simulink model "HoppingModel_Position"  (R2020a)
settings: Solver=FixedStepAuto  StartTime=0.0  StopTime=2  FixedStep=0.001  RelTol=1e-3
undefined symbols (not defined in the file or in its folder): chi_0, desired_energy, desired_energy2, desired_energy3, desired_energy4, desired_energy5, desired_energy6, desired_energy7, desired_energy8, g, H, H2, H3, H4, H5, H6, H7, H8, I1, I2, ini_theta1, ini_theta1_d, ini_theta2, ini_theta2_d, ini_w, ini_w_d, ini_x0, ini_x0_d, ini_x1, ini_x1_d, ini_x2, ini_x2_d, ini_y0, ini_y0_d, ini_y1, ini_y1_d, ini_y2, ini_y2_d, M1, M2, r1, r2, start_1, start_2, start_3, T2_change, T3_change, T4_change, T5_change, T6_change, T7_change, T8_change, x2_desired_1, x2_desired_2, x2_desired_3
settings Model: Creator=fabia  LastModifiedBy=fabia
settings DataIOCC: ReturnWorkspaceOutputs=off

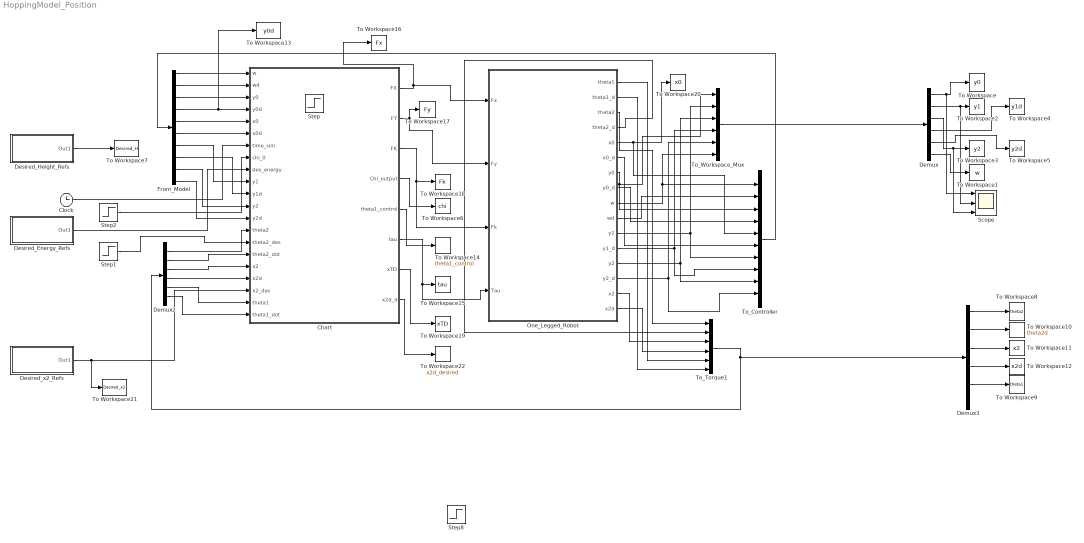
== system HoppingModel_Position ==
  Chart : Stateflow chart  TreatAsAtomicUnit=on
      settings: PortSchema="{\"entries\":[{\"content\":{\"sides\":[{\"content\":{\"connectorIds\":[\"In1\",\"In2\",\"In3\",\"In4\",\"In5\",\"In6\",\"In7\",\"In8\",\"In9\",\"In10\",\"In11\",\"In12\",\"In13\",\"In14\",\"In15\",\"In16\",\"In17\",\"In18\",\"In19\",\"In20\",\"In21\"]},\"type\":\"ConnectorPlacement.EquallySpacedRectSide\",\"uuid\":\"d60879a0-12a6-4ea9-8b3c-a4e8171fc461\"},{\"content\":{\"connectorIds\":[\"Out2\",\"Out1\",\"Out3\",\"Out4\",\"Out5\",\"Out6\",\"Out7\",\"Out8\"],\"side\":\"RIGHT\"},\"type\":\"ConnectorPlacement.EquallySpacedRectSide\",\"uuid\":\"e7f8c78b-f9da-45a1-b210-b73b1fe065f3\"},{\"content\":{\"connectorIds\":[],\"side\":\"TOP\"},\"type\":\"ConnectorPlacement.EquallySpacedRectSide\",\"uuid\":\"a7cfd386-52b0-4dd7-827b-34f43a49e5d2\"}]},\"type\":\"ConnectorPlacement.EquallySpacedConnector\",\"uuid\":\"c0fe03cd-cdd0-4cdb-8340-587840dec8d6\"}],\"packageUris\":[\"http://schema.mathworks.com/mf0/Connector/19700101\"],\"version\":\"1.0\"}"
  Clock : Clock
  Demux : Demux  Outputs=6
  Demux2 : Demux  Outputs=6
  Demux3 : Demux  Outputs=6
  Desired_Energy_Refs : Subsystem
  Desired_Height_Refs : Subsystem
  Desired_x2_Refs : Subsystem
  From_Model : Demux  Outputs=10
  One_Legged_Robot : Subsystem
  Scope : Scope  NumInputPorts=3
  Step : Step  Time=0  After=0  SampleTime=0
  Step1 : Step  Time=0  After=0  SampleTime=0
  Step2 : Step  Time=0  After=chi_0  SampleTime=0
  Step8 : Step  Time=T2_change  After=H2  SampleTime=0
  To Workspace : ToWorkspace  VariableName=y0  SaveFormat=Timeseries  SampleTime=-1
      settings: Save2DSignal=2-D array (concatenate along first dimension)
  To Workspace1 : ToWorkspace  VariableName=w  SaveFormat=Timeseries  SampleTime=-1
      settings: Save2DSignal=2-D array (concatenate along first dimension)
  To Workspace10 : ToWorkspace  VariableName=theta2d  SaveFormat=Timeseries  SampleTime=-1
      settings: Save2DSignal=2-D array (concatenate along first dimension)
  To Workspace11 : ToWorkspace  VariableName=x2  SaveFormat=Timeseries  SampleTime=-1
      settings: Save2DSignal=2-D array (concatenate along first dimension)
  To Workspace12 : ToWorkspace  VariableName=x2d  SaveFormat=Timeseries  SampleTime=-1
      settings: Save2DSignal=2-D array (concatenate along first dimension)
  To Workspace13 : ToWorkspace  VariableName=y0d  SaveFormat=Timeseries  SampleTime=-1
  To Workspace14 : ToWorkspace  VariableName=theta1_control  SaveFormat=Timeseries  SampleTime=-1
      settings: Save2DSignal=2-D array (concatenate along first dimension)
  To Workspace15 : ToWorkspace  VariableName=tau  SaveFormat=Timeseries  SampleTime=-1
      settings: Save2DSignal=2-D array (concatenate along first dimension)
  To Workspace16 : ToWorkspace  VariableName=Fx  SaveFormat=Timeseries  SampleTime=-1
      settings: Save2DSignal=2-D array (concatenate along first dimension)
  To Workspace17 : ToWorkspace  VariableName=Fy  SaveFormat=Timeseries  SampleTime=-1
      settings: Save2DSignal=2-D array (concatenate along first dimension)
  To Workspace18 : ToWorkspace  VariableName=Fk  SaveFormat=Timeseries  SampleTime=-1
      settings: Save2DSignal=2-D array (concatenate along first dimension)
  To Workspace19 : ToWorkspace  VariableName=xTD  SaveFormat=Timeseries  SampleTime=-1
      settings: Save2DSignal=2-D array (concatenate along first dimension)
  To Workspace2 : ToWorkspace  VariableName=y1  SaveFormat=Timeseries  SampleTime=-1
      settings: Save2DSignal=2-D array (concatenate along first dimension)
  To Workspace20 : ToWorkspace  VariableName=x0  SaveFormat=Timeseries  SampleTime=-1
      settings: Save2DSignal=2-D array (concatenate along first dimension)
  To Workspace21 : ToWorkspace  VariableName=Desired_x2  SaveFormat=Timeseries  SampleTime=-1
  To Workspace22 : ToWorkspace  VariableName=x2d_desired  SaveFormat=Timeseries  SampleTime=-1
      settings: Save2DSignal=2-D array (concatenate along first dimension)
  To Workspace3 : ToWorkspace  VariableName=y2  SaveFormat=Timeseries  SampleTime=-1
      settings: Save2DSignal=2-D array (concatenate along first dimension)
  To Workspace4 : ToWorkspace  VariableName=y1d  SaveFormat=Timeseries  SampleTime=-1
      settings: Save2DSignal=2-D array (concatenate along first dimension)
  To Workspace5 : ToWorkspace  VariableName=y2d  SaveFormat=Timeseries  SampleTime=-1
      settings: Save2DSignal=2-D array (concatenate along first dimension)
  To Workspace6 : ToWorkspace  VariableName=chi  SaveFormat=Timeseries  SampleTime=-1
      settings: Save2DSignal=2-D array (concatenate along first dimension)
  To Workspace7 : ToWorkspace  VariableName=Desired_H  SaveFormat=Timeseries  SampleTime=-1
  To Workspace8 : ToWorkspace  VariableName=theta2  SaveFormat=Timeseries  SampleTime=-1
      settings: Save2DSignal=2-D array (concatenate along first dimension)
  To Workspace9 : ToWorkspace  VariableName=theta1  SaveFormat=Timeseries  SampleTime=-1
      settings: Save2DSignal=2-D array (concatenate along first dimension)
  To_Controller : Mux  Inputs=10
  To_Torque1 : Mux  Inputs=6
  To_Workspace_Mux : Mux  Inputs=6
  wires:
  One_Legged_Robot/11(y1) -> To_Controller/7, To_Workspace_Mux/2
  One_Legged_Robot/13(y2) -> To_Controller/9, To_Workspace_Mux/3
  One_Legged_Robot/7(y0) -> To_Controller/3, To_Workspace_Mux/1
  One_Legged_Robot/5(x0) -> To Workspace20/1, To_Controller/5
  One_Legged_Robot/10(wd) -> To_Controller/2
  One_Legged_Robot/8(y0_d) -> To_Controller/4
  Chart/2(FX) -> One_Legged_Robot/1(Fx), To Workspace16/1
  Chart/1(FY) -> One_Legged_Robot/2(Fy), To Workspace17/1
  Chart/3(FK) -> To Workspace18/1, One_Legged_Robot/3(Fk)
  One_Legged_Robot/9(w) -> To_Workspace_Mux/6, To_Controller/1
  Clock/1 -> Chart/7(time_sim)
  Step2/1 -> Chart/8(chi_0)
  One_Legged_Robot/14(y2_d) -> To_Controller/10, To_Workspace_Mux/5
  Chart/4(Chi_output) -> To Workspace6/1
  One_Legged_Robot/6(x0_d) -> To_Controller/6
  One_Legged_Robot/12(y1_d) -> To_Controller/8, To_Workspace_Mux/4
  One_Legged_Robot/1(theta1) -> To_Torque1/5
  One_Legged_Robot/2(theta1_d) -> To_Torque1/6
  To_Controller/1 -> From_Model/1
  From_Model/1 -> Chart/1(w)
  From_Model/2 -> Chart/2(wd)
  From_Model/3 -> Chart/3(y0)
  From_Model/4 -> To Workspace13/1, Chart/4(y0d)
  From_Model/5 -> Chart/5(x0)
  From_Model/6 -> Chart/6(x0d)
  From_Model/7 -> Chart/10(y1)
  From_Model/8 -> Chart/11(y1d)
  From_Model/9 -> Chart/12(y2)
  From_Model/10 -> Chart/13(y2d)
  To_Workspace_Mux/1 -> Demux/1
  Demux/1 -> Scope/1, To Workspace/1
  Demux/2 -> Scope/2, To Workspace2/1
  Demux/3 -> Scope/3, To Workspace3/1
  Demux/4 -> To Workspace4/1
  Demux/5 -> To Workspace5/1
  Demux/6 -> To Workspace1/1
  Desired_Energy_Refs/1(Out1) -> Chart/9(des_energy)
  Desired_Height_Refs/1(Out1) -> To Workspace7/1
  One_Legged_Robot/3(theta2) -> To_Torque1/1
  One_Legged_Robot/4(theta2_d) -> To_Torque1/2
  One_Legged_Robot/15(x2) -> To_Torque1/3
  One_Legged_Robot/16(x2d) -> To_Torque1/4
  Demux2/1 -> Chart/14(theta2)
  Demux2/2 -> Chart/16(theta2_dot)
  Demux2/3 -> Chart/17(x2)
  Demux2/4 -> Chart/18(x2d)
  To_Torque1/1 -> Demux2/1, Demux3/1
  Chart/5(theta1_control) -> To Workspace14/1
  Step1/1 -> Chart/15(theta2_des)
  Demux3/4 -> To Workspace12/1
  Demux3/1 -> To Workspace8/1
  Demux3/3 -> To Workspace11/1
  Demux3/2 -> To Workspace10/1
  Demux3/5 -> To Workspace9/1
  Demux2/5 -> Chart/20(theta1)
  Demux2/6 -> Chart/21(theta1_dot)
  Chart/6(tau) -> One_Legged_Robot/4(Tau), To Workspace15/1
  Chart/7(xTD) -> To Workspace19/1
  Desired_x2_Refs/1(Out1) -> To Workspace21/1, Chart/19(x2_des)
  Chart/8(x2d_d) -> To Workspace22/1

== system HoppingModel_Position/Desired_Energy_Refs ==
  Add : Sum  Inputs=+-+-+-+-+-+-+-+
  Step1 : Step  Time=T3_change  After=desired_energy2  SampleTime=0
  Step10 : Step  Time=T6_change  After=desired_energy5  SampleTime=0
  Step11 : Step  Time=T6_change  After=desired_energy6  SampleTime=0
  Step12 : Step  Time=T7_change  After=desired_energy6  SampleTime=0
  Step13 : Step  Time=T7_change  After=desired_energy7  SampleTime=0
  Step14 : Step  Time=T8_change  After=desired_energy7  SampleTime=0
  Step15 : Step  Time=T8_change  After=desired_energy8  SampleTime=0
  Step2 : Step  Time=T3_change  After=desired_energy3  SampleTime=0
  Step3 : Step  Time=T4_change  After=desired_energy3  SampleTime=0
  Step4 : Step  Time=0  After=desired_energy  SampleTime=0
  Step5 : Step  Time=T2_change  After=desired_energy  SampleTime=0
  Step6 : Step  Time=T2_change  After=desired_energy2  SampleTime=0
  Step7 : Step  Time=T4_change  After=desired_energy4  SampleTime=0
  Step8 : Step  Time=T5_change  After=desired_energy4  SampleTime=0
  Step9 : Step  Time=T5_change  After=desired_energy5  SampleTime=0
  Out1 : Outport
  wires:
  Step6/1 -> Add/3
  Step4/1 -> Add/1
  Step5/1 -> Add/2
  Add/1 -> Out1/1
  Step1/1 -> Add/4
  Step2/1 -> Add/5
  Step3/1 -> Add/6
  Step7/1 -> Add/7
  Step8/1 -> Add/8
  Step9/1 -> Add/9
  Step10/1 -> Add/10
  Step11/1 -> Add/11
  Step12/1 -> Add/12
  Step13/1 -> Add/13
  Step14/1 -> Add/14
  Step15/1 -> Add/15

== system HoppingModel_Position/Desired_Height_Refs ==
  Add : Sum  Inputs=+-+-+-+-+-+-+-+
  Step1 : Step  Time=T3_change  After=H2  SampleTime=0
  Step10 : Step  Time=T6_change  After=H5  SampleTime=0
  Step11 : Step  Time=T6_change  After=H6  SampleTime=0
  Step12 : Step  Time=T7_change  After=H6  SampleTime=0
  Step13 : Step  Time=T7_change  After=H7  SampleTime=0
  Step14 : Step  Time=T8_change  After=H7  SampleTime=0
  Step15 : Step  Time=T8_change  After=H8  SampleTime=0
  Step2 : Step  Time=T3_change  After=H3  SampleTime=0
  Step3 : Step  Time=T4_change  After=H3  SampleTime=0
  Step4 : Step  Time=0  After=H  SampleTime=0
  Step5 : Step  Time=T2_change  After=H  SampleTime=0
  Step6 : Step  Time=T2_change  After=H2  SampleTime=0
  Step7 : Step  Time=T4_change  After=H4  SampleTime=0
  Step8 : Step  Time=T5_change  After=H4  SampleTime=0
  Step9 : Step  Time=T5_change  After=H5  SampleTime=0
  Out1 : Outport
  wires:
  Step6/1 -> Add/3
  Step4/1 -> Add/1
  Step5/1 -> Add/2
  Add/1 -> Out1/1
  Step1/1 -> Add/4
  Step2/1 -> Add/5
  Step3/1 -> Add/6
  Step7/1 -> Add/7
  Step8/1 -> Add/8
  Step9/1 -> Add/9
  Step10/1 -> Add/10
  Step11/1 -> Add/11
  Step12/1 -> Add/12
  Step13/1 -> Add/13
  Step14/1 -> Add/14
  Step15/1 -> Add/15

== system HoppingModel_Position/Desired_x2_Refs ==
  Add : Sum  Inputs=+-+-+
  Step1 : Step  Time=start_2  After=x2_desired_1  SampleTime=0
  Step2 : Step  Time=start_3  After=x2_desired_2  SampleTime=0
  Step3 : Step  Time=start_3  After=x2_desired_3  SampleTime=0
  Step4 : Step  Time=start_1  After=x2_desired_1  SampleTime=0
  Step6 : Step  Time=start_2  After=x2_desired_2  SampleTime=0
  Out1 : Outport
  wires:
  Step6/1 -> Add/3
  Step4/1 -> Add/1
  Step1/1 -> Add/2
  Add/1 -> Out1/1
  Step2/1 -> Add/4
  Step3/1 -> Add/5

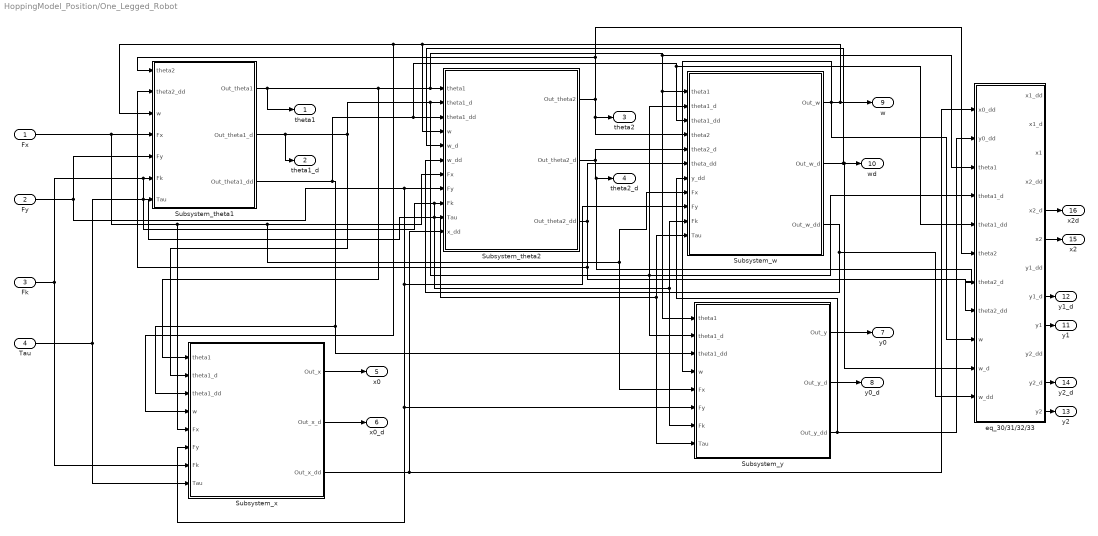
== system HoppingModel_Position/One_Legged_Robot ==
  Fx : Inport
  Fy : Inport  Port=2
  Fk : Inport  Port=3
  Tau : Inport  Port=4
  Subsystem_theta1 : Subsystem
  Subsystem_theta2 : Subsystem
  Subsystem_w : Subsystem
  Subsystem_x : Subsystem
  Subsystem_y : Subsystem
  "eq_30/31/32/33 " : Subsystem
  theta1 : Outport
  theta1_d : Outport  Port=2
  theta2 : Outport  Port=3
  theta2_d : Outport  Port=4
  x0 : Outport  Port=5
  x0_d : Outport  Port=6
  y0 : Outport  Port=7
  y0_d : Outport  Port=8
  w : Outport  Port=9
  wd : Outport  Port=10
  y1 : Outport  Port=11
  y1_d : Outport  Port=12
  y2 : Outport  Port=13
  y2_d : Outport  Port=14
  x2 : Outport  Port=15
  x2d : Outport  Port=16
  wires:
  Subsystem_theta1/1(Out_theta1) -> Subsystem_x/1(theta1), "eq_30/31/32/33 "/3(theta1), Subsystem_y/1(theta1), Subsystem_w/1(theta1), Subsystem_theta2/1(theta1), theta1/1
  Subsystem_theta1/2(Out_theta1_d) -> Subsystem_y/2(theta1_d), "eq_30/31/32/33 "/4(theta1_d), Subsystem_w/2(theta1_d), Subsystem_theta2/2(theta1_d), Subsystem_x/2(theta1_d), theta1_d/1
  Subsystem_x/1(Out_x) -> x0/1
  Subsystem_x/2(Out_x_d) -> x0_d/1
  Subsystem_y/1(Out_y) -> y0/1
  Subsystem_y/2(Out_y_d) -> y0_d/1
  "eq_30/31/32/33 "/9(y1) -> y1/1
  "eq_30/31/32/33 "/8(y1_d) -> y1_d/1
  "eq_30/31/32/33 "/12(y2) -> y2/1
  "eq_30/31/32/33 "/11(y2_d) -> y2_d/1
  Subsystem_w/2(Out_w_d) -> "eq_30/31/32/33 "/10(w_d), wd/1, Subsystem_theta2/5(w_d)
  Subsystem_w/1(Out_w) -> Subsystem_y/4(w), "eq_30/31/32/33 "/9(w), Subsystem_theta2/4(w), Subsystem_x/4(w), Subsystem_theta1/3(w), w/1
  Subsystem_theta2/1(Out_theta2) -> "eq_30/31/32/33 "/6(theta2), Subsystem_theta1/1(theta2), Subsystem_w/4(theta2), theta2/1
  Subsystem_theta2/2(Out_theta2_d) -> Subsystem_w/5(theta2_d), "eq_30/31/32/33 "/7(theta2_d), theta2_d/1
  Subsystem_theta1/3(Out_theta1_dd) -> Subsystem_x/3(theta1_dd), Subsystem_y/3(theta1_dd), "eq_30/31/32/33 "/5(theta1_dd), Subsystem_w/3(theta1_dd), Subsystem_theta2/3(theta1_dd)
  Subsystem_theta2/3(Out_theta2_dd) -> "eq_30/31/32/33 "/8(theta2_dd), Subsystem_theta1/2(theta2_dd), Subsystem_w/6(theta_dd)
  Subsystem_w/3(Out_w_dd) -> "eq_30/31/32/33 "/11(w_dd), Subsystem_theta2/6(w_dd)
  Subsystem_y/3(Out_y_dd) -> "eq_30/31/32/33 "/2(y0_dd), Subsystem_w/7(y_dd)
  Subsystem_x/3(Out_x_dd) -> "eq_30/31/32/33 "/1(x0_dd), Subsystem_theta2/11(x_dd)
  Fx/1 -> Subsystem_x/5(Fx), Subsystem_y/5(Fx), Subsystem_w/8(Fx), Subsystem_theta2/7(Fx), Subsystem_theta1/4(Fx)
  Fy/1 -> Subsystem_w/9(Fy), Subsystem_x/6(Fy), Subsystem_y/6(Fy), Subsystem_theta2/8(Fy), Subsystem_theta1/5(Fy)
  Fk/1 -> Subsystem_x/7(Fk), Subsystem_y/7(Fk), Subsystem_w/10(Fk), Subsystem_theta2/9(Fk), Subsystem_theta1/6(Fk)
  Tau/1 -> Subsystem_x/8(Tau), Subsystem_y/8(Tau), Subsystem_w/11(Tau), Subsystem_theta2/10(Tau), Subsystem_theta1/7(Tau)
  "eq_30/31/32/33 "/6(x2) -> x2/1
  "eq_30/31/32/33 "/5(x2_d) -> x2d/1

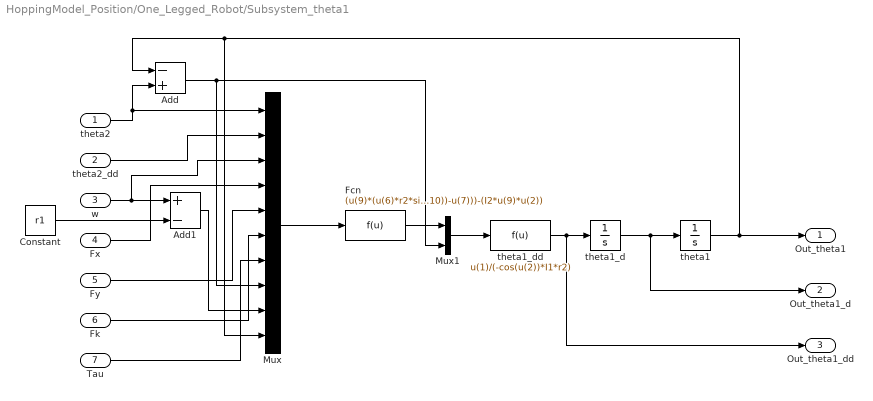
== system HoppingModel_Position/One_Legged_Robot/Subsystem_theta1 ==
  theta2 : Inport
  theta2_dd : Inport  Port=2
  w : Inport  Port=3
  Fx : Inport  Port=4
  Fy : Inport  Port=5
  Fk : Inport  Port=6
  Tau : Inport  Port=7
  Add : Sum  Inputs=-+
  Add1 : Sum  Inputs=+-
  Constant : Constant  Value=r1
  Fcn : Fcn  Expr=(u(9)*(u(6)*r2*sin(u(8))+u(7)))-(r2*cos(u(8))*(r1*u(5)*sin(u(10))-r1*u(4)*cos(u(10))-u(7)))-(I2*u(9)*u(2))
  Mux : Mux  Inputs=10
  Mux1 : Mux  Inputs=2
  theta1 : Integrator  InitialCondition=ini_theta1  UpperSaturationLimit=pi/2  LowerSaturationLimit=-pi/2
  theta1_d : Integrator  InitialCondition=ini_theta1_d  UpperSaturationLimit=pi/2  LowerSaturationLimit=-pi/2
  theta1_dd : Fcn  Expr=u(1)/(-cos(u(2))*I1*r2)
  Out_theta1 : Outport
  Out_theta1_d : Outport  Port=2
  Out_theta1_dd : Outport  Port=3
  wires:
  theta2/1 -> Mux/1, Add/2
  theta1/1 -> Out_theta1/1, Mux/10, Add/1
  w/1 -> Mux/3, Add1/1
  Constant/1 -> Add1/2
  theta2_dd/1 -> Mux/2
  Fx/1 -> Mux/4
  Fy/1 -> Mux/5
  Fk/1 -> Mux/6
  Tau/1 -> Mux/7
  Add/1 -> Mux/8, Mux1/2
  Add1/1 -> Mux/9
  Mux/1 -> Fcn/1
  Fcn/1 -> Mux1/1
  Mux1/1 -> theta1_dd/1
  theta1_dd/1 -> Out_theta1_dd/1, theta1_d/1
  theta1_d/1 -> Out_theta1_d/1, theta1/1

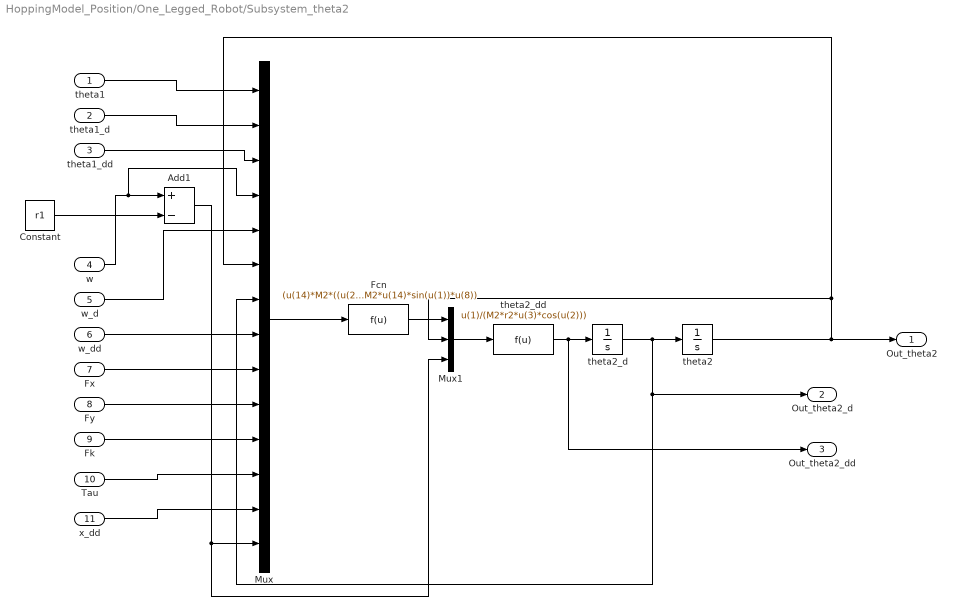
== system HoppingModel_Position/One_Legged_Robot/Subsystem_theta2 ==
  theta1 : Inport
  theta1_d : Inport  Port=2
  theta1_dd : Inport  Port=3
  w : Inport  Port=4
  w_d : Inport  Port=5
  w_dd : Inport  Port=6
  Fx : Inport  Port=7
  Fy : Inport  Port=8
  Fk : Inport  Port=9
  Tau : Inport  Port=10
  x_dd : Inport  Port=11
  Add1 : Sum  Inputs=+-
  Constant : Constant  Value=r1
  Fcn : Fcn  Expr=(u(14)*M2*((u(2)^2)*u(14)*sin(u(1))-2*u(2)*u(5)*cos(u(1))+r2*(u(7)^2)*sin(u(6))+r1*(u(2)^2)*sin(u(1))))-(r1*u(9)*(cos(u(1)))^2)+(cos(u(1))*(r1*u(10)*sin(u(1))-u(12)))+(u(11)*u(14)*sin(u(1)))-(M2*u(14)*u(13))-(cos(u(1))*(M2*u(14)*u(4)+I1)*u(3))-(M2*u(14)*sin(u(1))*u(8))
  Mux : Mux  Inputs=14
  Mux1 : Mux  Inputs=3
  theta2 : Integrator  InitialCondition=ini_theta2
  theta2_d : Integrator  InitialCondition=ini_theta2_d
  theta2_dd : Fcn  Expr=u(1)/(M2*r2*u(3)*cos(u(2)))
  Out_theta2 : Outport
  Out_theta2_d : Outport  Port=2
  Out_theta2_dd : Outport  Port=3
  wires:
  Fcn/1 -> Mux1/1
  Mux1/1 -> theta2_dd/1
  theta2_dd/1 -> Out_theta2_dd/1, theta2_d/1
  theta2_d/1 -> Mux/7, Out_theta2_d/1, theta2/1
  Constant/1 -> Add1/2
  theta1/1 -> Mux/1
  theta1_d/1 -> Mux/2
  theta1_dd/1 -> Mux/3
  Add1/1 -> Mux1/3, Mux/14
  Mux/1 -> Fcn/1
  w/1 -> Mux/4, Add1/1
  w_d/1 -> Mux/5
  w_dd/1 -> Mux/8
  Fx/1 -> Mux/9
  Fy/1 -> Mux/10
  Fk/1 -> Mux/11
  Tau/1 -> Mux/12
  x_dd/1 -> Mux/13
  theta2/1 -> Mux/6, Mux1/2, Out_theta2/1

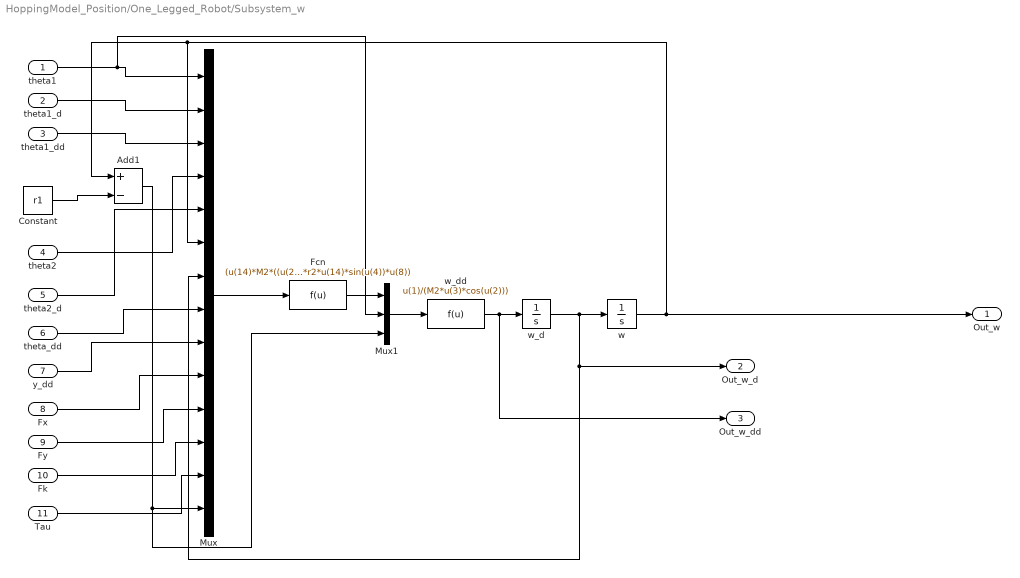
== system HoppingModel_Position/One_Legged_Robot/Subsystem_w ==
  theta1 : Inport
  theta1_d : Inport  Port=2
  theta1_dd : Inport  Port=3
  theta2 : Inport  Port=4
  theta2_d : Inport  Port=5
  theta_dd : Inport  Port=6
  y_dd : Inport  Port=7
  Fx : Inport  Port=8
  Fy : Inport  Port=9
  Fk : Inport  Port=10
  Tau : Inport  Port=11
  Add1 : Sum  Inputs=+-
  Constant : Constant  Value=r1
  Fcn : Fcn  Expr=(u(14)*M2*((u(2)^2)*u(14)*cos(u(1))+2*u(2)*u(7)*sin(u(1))+r2*(u(5)^2)*cos(u(4))+r1*(u(2)^2)*cos(u(1))-g))+(r1*u(10)*cos(u(1))*sin(u(1)))-(sin(u(1))*(r1*u(11)*sin(u(1))-u(13)))+(u(12)*u(14)*cos(u(1)))+(sin(u(1))*(M2*u(14)*u(6)+I1)*u(3))-(M2*u(14)*u(9))+(M2*r2*u(14)*sin(u(4))*u(8))
  Mux : Mux  Inputs=14
  Mux1 : Mux  Inputs=3
  w : Integrator  InitialCondition=ini_w
  w_d : Integrator  InitialCondition=ini_w_d
  w_dd : Fcn  Expr=u(1)/(M2*u(3)*cos(u(2)))
  Out_w : Outport
  Out_w_d : Outport  Port=2
  Out_w_dd : Outport  Port=3
  wires:
  Fcn/1 -> Mux1/1
  Mux1/1 -> w_dd/1
  w_dd/1 -> Out_w_dd/1, w_d/1
  w_d/1 -> Mux/7, Out_w_d/1, w/1
  Constant/1 -> Add1/2
  Mux/1 -> Fcn/1
  Add1/1 -> Mux1/3, Mux/14
  theta1/1 -> Mux1/2, Mux/1
  theta1_d/1 -> Mux/2
  theta1_dd/1 -> Mux/3
  theta2/1 -> Mux/4
  theta2_d/1 -> Mux/5
  theta_dd/1 -> Mux/8
  y_dd/1 -> Mux/9
  Fx/1 -> Mux/10
  Fy/1 -> Mux/11
  Fk/1 -> Mux/12
  Tau/1 -> Mux/13
  w/1 -> Mux/6, Add1/1, Out_w/1

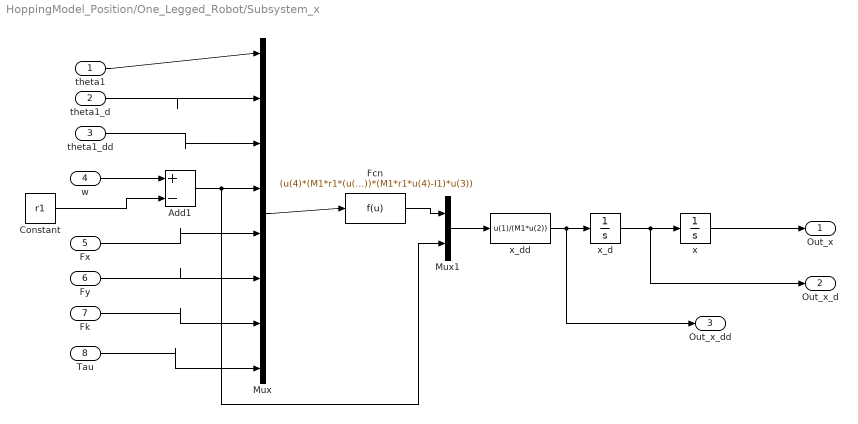
== system HoppingModel_Position/One_Legged_Robot/Subsystem_x ==
  theta1 : Inport
  theta1_d : Inport  Port=2
  theta1_dd : Inport  Port=3
  w : Inport  Port=4
  Fx : Inport  Port=5
  Fy : Inport  Port=6
  Fk : Inport  Port=7
  Tau : Inport  Port=8
  Add1 : Sum  Inputs=+-
  Constant : Constant  Value=r1
  Fcn : Fcn  Expr=(u(4)*(M1*r1*(u(2)^2)*sin(u(1))-u(7)*sin(u(1))+u(5)))-(cos(u(1))*(u(6)*r1*sin(u(1))-u(5)*r1*cos(u(1))-u(8)))-(cos(u(1))*(M1*r1*u(4)-I1)*u(3))
  Mux : Mux  Inputs=8
  Mux1 : Mux  Inputs=2
  x : Integrator  InitialCondition=ini_x0
  x_d : Integrator  InitialCondition=ini_x0_d
  x_dd : Fcn  Expr=u(1)/(M1*u(2))
  Out_x : Outport
  Out_x_d : Outport  Port=2
  Out_x_dd : Outport  Port=3
  wires:
  x/1 -> Out_x/1
  Fcn/1 -> Mux1/1
  Mux1/1 -> x_dd/1
  x_dd/1 -> Out_x_dd/1, x_d/1
  x_d/1 -> Out_x_d/1, x/1
  Constant/1 -> Add1/2
  Mux/1 -> Fcn/1
  w/1 -> Add1/1
  theta1/1 -> Mux/1
  theta1_d/1 -> Mux/2
  theta1_dd/1 -> Mux/3
  Add1/1 -> Mux1/2, Mux/4
  Fx/1 -> Mux/5
  Fy/1 -> Mux/6
  Fk/1 -> Mux/7
  Tau/1 -> Mux/8

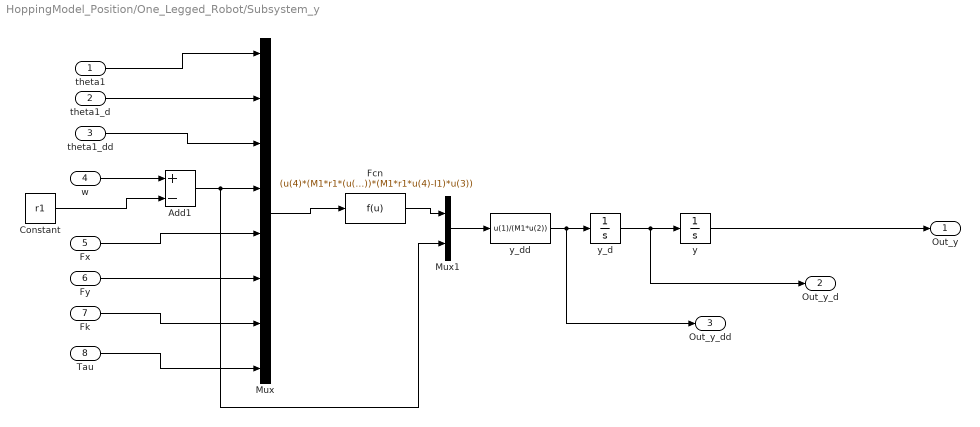
== system HoppingModel_Position/One_Legged_Robot/Subsystem_y ==
  theta1 : Inport
  theta1_d : Inport  Port=2
  theta1_dd : Inport  Port=3
  w : Inport  Port=4
  Fx : Inport  Port=5
  Fy : Inport  Port=6
  Fk : Inport  Port=7
  Tau : Inport  Port=8
  Add1 : Sum  Inputs=+-
  Constant : Constant  Value=r1
  Fcn : Fcn  Expr=(u(4)*(M1*r1*(u(2)^2)*cos(u(1))-u(7)*cos(u(1))+u(6)-M1*g))+(sin(u(1))*(u(6)*r1*sin(u(1))-u(5)*r1*cos(u(1))-u(8)))+(sin(u(1))*(M1*r1*u(4)-I1)*u(3))
  Mux : Mux  Inputs=8
  Mux1 : Mux  Inputs=2
  y : Integrator  InitialCondition=ini_y0
  y_d : Integrator  InitialCondition=ini_y0_d
  y_dd : Fcn  Expr=u(1)/(M1*u(2))
  Out_y : Outport
  Out_y_d : Outport  Port=2
  Out_y_dd : Outport  Port=3
  wires:
  Fcn/1 -> Mux1/1
  Mux1/1 -> y_dd/1
  y_dd/1 -> Out_y_dd/1, y_d/1
  y_d/1 -> Out_y_d/1, y/1
  Constant/1 -> Add1/2
  Mux/1 -> Fcn/1
  w/1 -> Add1/1
  theta1/1 -> Mux/1
  theta1_d/1 -> Mux/2
  theta1_dd/1 -> Mux/3
  Add1/1 -> Mux1/2, Mux/4
  Fx/1 -> Mux/5
  Fy/1 -> Mux/6
  Fk/1 -> Mux/7
  Tau/1 -> Mux/8
  y/1 -> Out_y/1

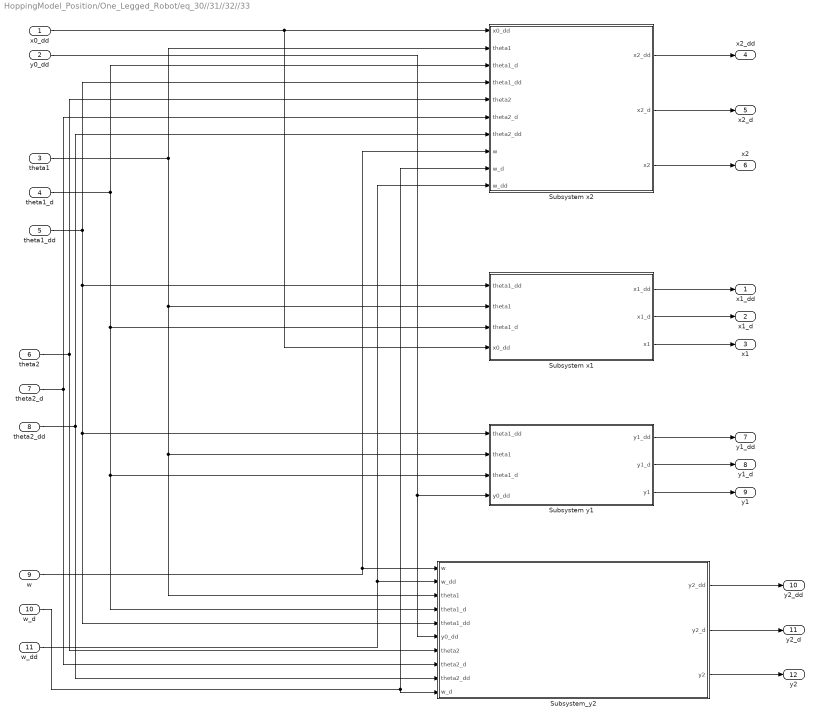
== system HoppingModel_Position/One_Legged_Robot/eq_30//31//32//33  ==
  x0_dd : Inport
  y0_dd : Inport  Port=2
  theta1 : Inport  Port=3
  theta1_d : Inport  Port=4
  theta1_dd : Inport  Port=5
  theta2 : Inport  Port=6
  theta2_d : Inport  Port=7
  theta2_dd : Inport  Port=8
  w : Inport  Port=9
  w_d : Inport  Port=10
  w_dd : Inport  Port=11
  Subsystem x1 : Subsystem
  Subsystem x2 : Subsystem
  Subsystem y1 : Subsystem
  Subsystem_y2 : Subsystem
  x1_dd : Outport
  x1_d : Outport  Port=2
  x1 : Outport  Port=3
  x2_dd : Outport  Port=4
  x2_d : Outport  Port=5
  x2 : Outport  Port=6
  y1_dd : Outport  Port=7
  y1_d : Outport  Port=8
  y1 : Outport  Port=9
  y2_dd : Outport  Port=10
  y2_d : Outport  Port=11
  y2 : Outport  Port=12
  wires:
  Subsystem x1/1(x1_dd) -> x1_dd/1
  Subsystem x1/3(x1) -> x1/1
  x0_dd/1 -> Subsystem x1/4(x0_dd), Subsystem x2/1(x0_dd)
  Subsystem_y2/1(y2_dd) -> y2_dd/1
  theta1_d/1 -> Subsystem_y2/4(theta1_d), Subsystem y1/3(theta1_d), Subsystem x1/3(theta1_d), Subsystem x2/3(theta1_d)
  Subsystem x2/1(x2_dd) -> x2_dd/1
  Subsystem x2/3(x2) -> x2/1
  w_dd/1 -> Subsystem x2/10(w_dd), Subsystem_y2/2(w_dd)
  Subsystem_y2/3(y2) -> y2/1
  theta1/1 -> Subsystem_y2/3(theta1), Subsystem y1/2(theta1), Subsystem x1/2(theta1), Subsystem x2/2(theta1)
  Subsystem x1/2(x1_d) -> x1_d/1
  theta1_dd/1 -> Subsystem_y2/5(theta1_dd), Subsystem y1/1("theta1_dd "), Subsystem x1/1("theta1_dd "), Subsystem x2/4(theta1_dd)
  y0_dd/1 -> Subsystem_y2/6(y0_dd), Subsystem y1/4(y0_dd)
  theta2_dd/1 -> Subsystem x2/7("theta2_dd "), Subsystem_y2/9(theta2_dd)
  w_d/1 -> Subsystem_y2/10(w_d), Subsystem x2/9(w_d)
  Subsystem x2/2(x2_d) -> x2_d/1
  Subsystem y1/3(y1) -> y1/1
  theta2_d/1 -> Subsystem x2/6(theta2_d), Subsystem_y2/8(theta2_d)
  theta2/1 -> Subsystem x2/5(theta2), Subsystem_y2/7(theta2)
  w/1 -> Subsystem x2/8(w), Subsystem_y2/1(w)
  Subsystem y1/2(y1_d) -> y1_d/1
  Subsystem y1/1(y1_dd) -> y1_dd/1
  Subsystem_y2/2(y2_d) -> y2_d/1

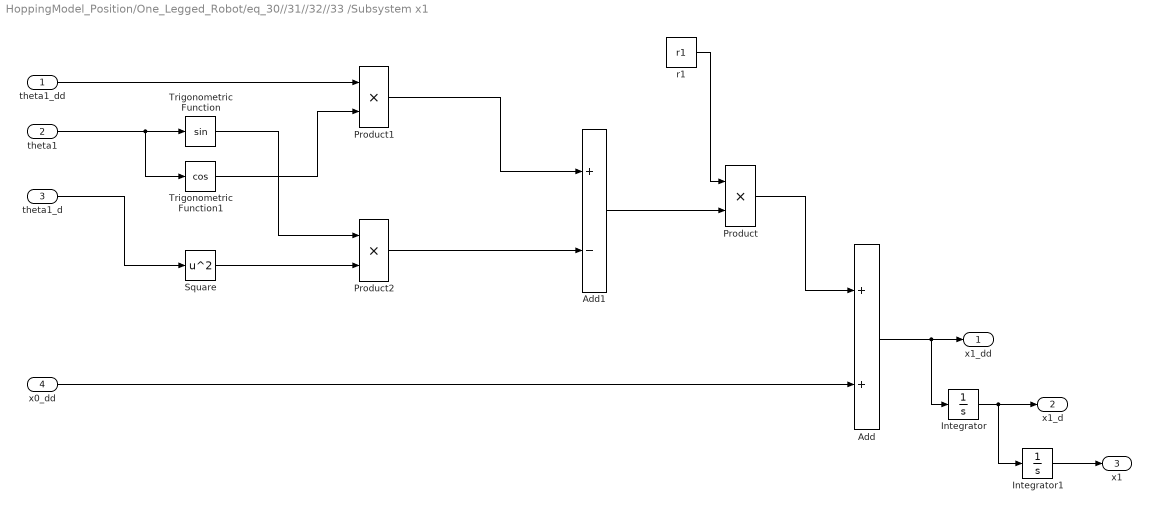
== system HoppingModel_Position/One_Legged_Robot/eq_30//31//32//33 /Subsystem x1 ==
  "theta1_dd " : Inport
  theta1 : Inport  Port=2
  theta1_d : Inport  Port=3
  x0_dd : Inport  Port=4
  Add : Sum
  Add1 : Sum  Inputs=+-
  Integrator : Integrator  InitialCondition=ini_x1_d
  Integrator1 : Integrator  InitialCondition=ini_x1
  Product : Product
  Product1 : Product
  Product2 : Product
  Square : Math  Operator=square  SaturateOnIntegerOverflow=on
  Trigonometric Function : Trigonometry
  Trigonometric Function1 : Trigonometry  Operator=cos
  r1 : Constant  Value=r1
  x1_dd : Outport
  x1_d : Outport  Port=2
  x1 : Outport  Port=3
  wires:
  Add1/1 -> Product/2
  Product/1 -> Add/1
  Product2/1 -> Add1/2
  r1/1 -> Product/1
  Trigonometric Function1/1 -> Product1/2
  x0_dd/1 -> Add/2
  theta1_d/1 -> Square/1
  Trigonometric Function/1 -> Product2/1
  Integrator/1 -> x1_d/1, Integrator1/1
  Add/1 -> x1_dd/1, Integrator/1
  Square/1 -> Product2/2
  Product1/1 -> Add1/1
  "theta1_dd "/1 -> Product1/1
  theta1/1 -> Trigonometric Function1/1, Trigonometric Function/1
  Integrator1/1 -> x1/1

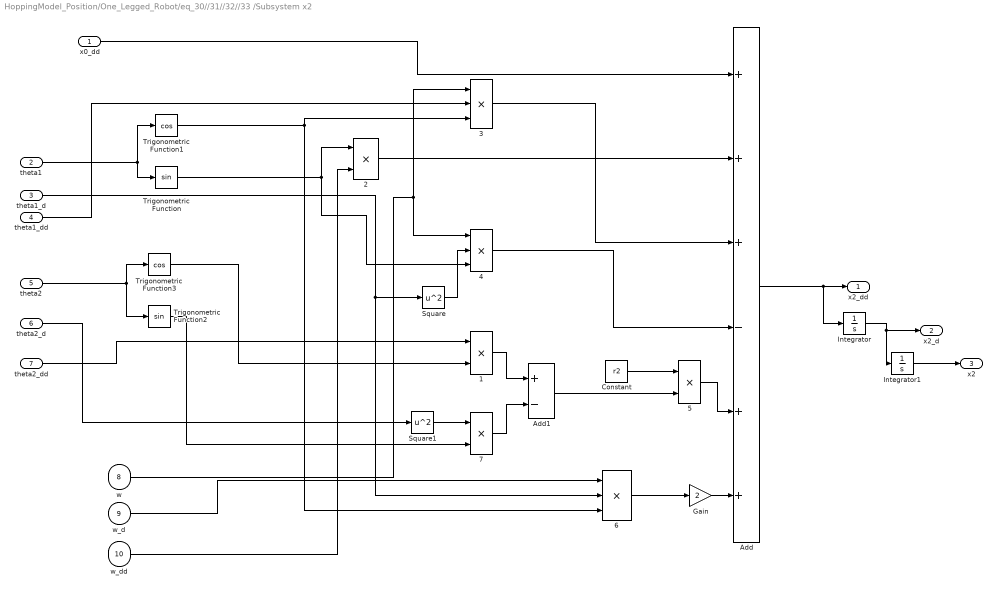
== system HoppingModel_Position/One_Legged_Robot/eq_30//31//32//33 /Subsystem x2 ==
  x0_dd : Inport
  theta1 : Inport  Port=2
  theta1_d : Inport  Port=3
  theta1_dd : Inport  Port=4
  theta2 : Inport  Port=5
  theta2_d : Inport  Port=6
  "theta2_dd " : Inport  Port=7
  w : Inport  Port=8
  w_d : Inport  Port=9
  w_dd : Inport  Port=10
  {1..2,5,7} (4 alike) : Product
  3 : Product  Inputs=3
  4 : Product  Inputs=3
  6 : Product  Inputs=3
  Add : Sum  Inputs=+++-++
  Add1 : Sum  Inputs=+-
  Constant : Constant  Value=r2
  Gain : Gain  Gain=2
  Integrator : Integrator  InitialCondition=ini_x2_d
  Integrator1 : Integrator  InitialCondition=ini_x2
  Square : Math  Operator=square  SaturateOnIntegerOverflow=on
  Square1 : Math  Operator=square  SaturateOnIntegerOverflow=on
  Trigonometric Function : Trigonometry
  Trigonometric Function1 : Trigonometry  Operator=cos
  Trigonometric Function2 : Trigonometry
  Trigonometric Function3 : Trigonometry  Operator=cos
  x2_dd : Outport
  x2_d : Outport  Port=2
  x2 : Outport  Port=3
  wires:
  7/1 -> Add1/2
  Integrator1/1 -> x2/1
  w_d/1 -> 6/1
  Constant/1 -> 5/1
  Integrator/1 -> x2_d/1, Integrator1/1
  Trigonometric Function1/1 -> 6/3, 3/3
  x0_dd/1 -> Add/1
  Add1/1 -> 5/2
  theta2/1 -> Trigonometric Function3/1, Trigonometric Function2/1
  6/1 -> Gain/1
  4/1 -> Add/4
  Square/1 -> 4/2
  theta1_d/1 -> 6/2, Square/1
  Square1/1 -> 7/1
  w/1 -> 3/1, 4/1
  Add/1 -> x2_dd/1, Integrator/1
  Trigonometric Function2/1 -> 7/2
  Trigonometric Function3/1 -> 1/2
  w_dd/1 -> 2/2
  theta1/1 -> Trigonometric Function1/1, Trigonometric Function/1
  Gain/1 -> Add/6
  Trigonometric Function/1 -> 4/3, 2/1
  theta1_dd/1 -> 3/2
  3/1 -> Add/3
  1/1 -> Add1/1
  2/1 -> Add/2
  5/1 -> Add/5
  "theta2_dd "/1 -> 1/1
  theta2_d/1 -> Square1/1

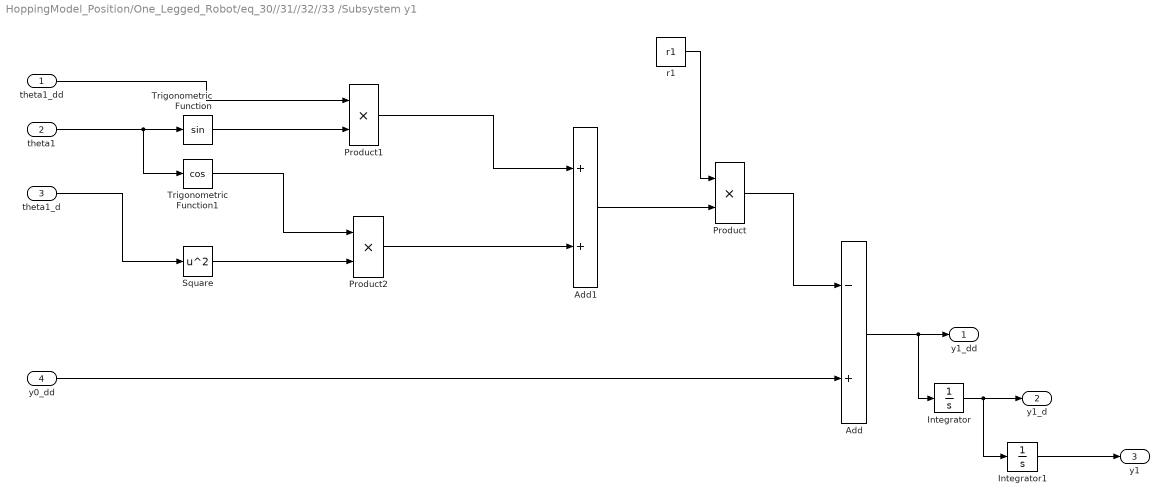
== system HoppingModel_Position/One_Legged_Robot/eq_30//31//32//33 /Subsystem y1 ==
  "theta1_dd " : Inport
  theta1 : Inport  Port=2
  theta1_d : Inport  Port=3
  y0_dd : Inport  Port=4
  Add : Sum  Inputs=-+
  Add1 : Sum
  Integrator : Integrator  InitialCondition=ini_y1_d
  Integrator1 : Integrator  InitialCondition=ini_y1
  Product : Product
  Product1 : Product
  Product2 : Product
  Square : Math  Operator=square  SaturateOnIntegerOverflow=on
  Trigonometric Function : Trigonometry
  Trigonometric Function1 : Trigonometry  Operator=cos
  r1 : Constant  Value=r1
  y1_dd : Outport
  y1_d : Outport  Port=2
  y1 : Outport  Port=3
  wires:
  "theta1_dd "/1 -> Product1/1
  Product1/1 -> Add1/1
  y0_dd/1 -> Add/2
  Integrator/1 -> y1_d/1, Integrator1/1
  Add/1 -> y1_dd/1, Integrator/1
  r1/1 -> Product/1
  Integrator1/1 -> y1/1
  theta1/1 -> Trigonometric Function1/1, Trigonometric Function/1
  Square/1 -> Product2/2
  theta1_d/1 -> Square/1
  Product/1 -> Add/1
  Trigonometric Function/1 -> Product1/2
  Product2/1 -> Add1/2
  Add1/1 -> Product/2
  Trigonometric Function1/1 -> Product2/1

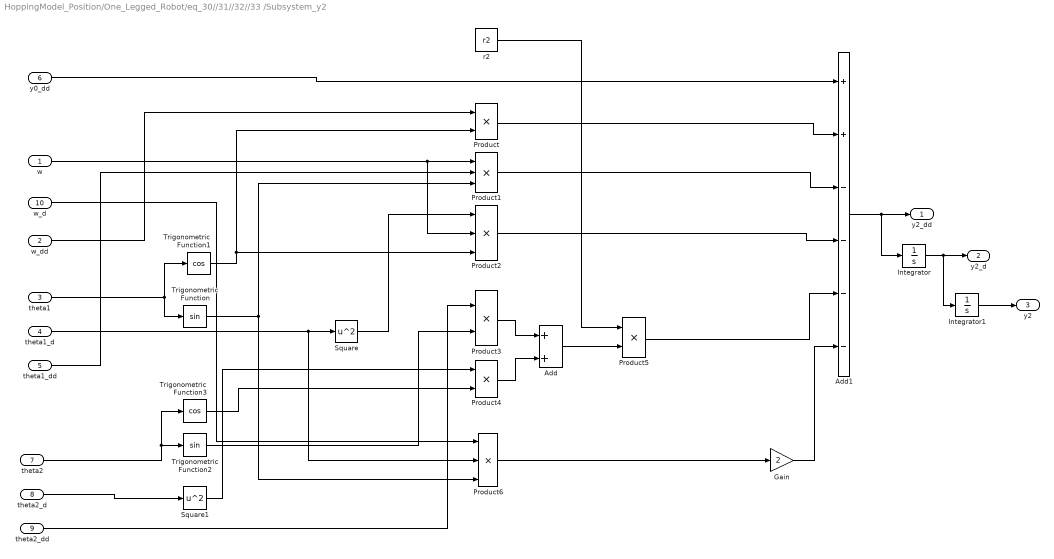
== system HoppingModel_Position/One_Legged_Robot/eq_30//31//32//33 /Subsystem_y2 ==
  w : Inport
  w_dd : Inport  Port=2
  theta1 : Inport  Port=3
  theta1_d : Inport  Port=4
  theta1_dd : Inport  Port=5
  y0_dd : Inport  Port=6
  theta2 : Inport  Port=7
  theta2_d : Inport  Port=8
  theta2_dd : Inport  Port=9
  w_d : Inport  Port=10
  Add : Sum
  Add1 : Sum  Inputs=++----
  Gain : Gain  Gain=2
  Integrator : Integrator  InitialCondition=ini_y2_d
  Integrator1 : Integrator  InitialCondition=ini_y2
  Product{,3..5} (4 alike) : Product
  Product1 : Product  Inputs=3
  Product2 : Product  Inputs=3
  Product6 : Product  Inputs=3
  Square : Math  Operator=square  SaturateOnIntegerOverflow=on
  Square1 : Math  Operator=square  SaturateOnIntegerOverflow=on
  Trigonometric Function : Trigonometry
  Trigonometric Function1 : Trigonometry  Operator=cos
  Trigonometric Function2 : Trigonometry
  Trigonometric Function3 : Trigonometry  Operator=cos
  r2 : Constant  Value=r2
  y2_dd : Outport
  y2_d : Outport  Port=2
  y2 : Outport  Port=3
  wires:
  r2/1 -> Product5/1
  Product2/1 -> Add1/4
  theta2_d/1 -> Square1/1
  Product5/1 -> Add1/5
  Product1/1 -> Add1/3
  y0_dd/1 -> Add1/1
  Product3/1 -> Add/1
  Product6/1 -> Gain/1
  theta1_d/1 -> Product6/2, Square/1
  Integrator1/1 -> y2/1
  w/1 -> Product2/2, Product1/1
  Trigonometric Function/1 -> Product1/3, Product6/3
  theta1_dd/1 -> Product1/2
  Integrator/1 -> y2_d/1, Integrator1/1
  Product/1 -> Add1/2
  w_d/1 -> Product6/1
  theta1/1 -> Trigonometric Function1/1, Trigonometric Function/1
  w_dd/1 -> Product/1
  Gain/1 -> Add1/6
  Trigonometric Function1/1 -> Product/2, Product2/3
  Square1/1 -> Product4/1
  theta2/1 -> Trigonometric Function3/1, Trigonometric Function2/1
  Add1/1 -> y2_dd/1, Integrator/1
  Product4/1 -> Add/2
  Trigonometric Function2/1 -> Product3/2
  Trigonometric Function3/1 -> Product4/2
  Add/1 -> Product5/2
  Square/1 -> Product2/1
  theta2_dd/1 -> Product3/1

== stateflow chart HoppingModel_Position/Chart ==
  settings: updateMethod=DISCRETE  sampleTime=0.001
  state Bottom_LiftOff
    entry:
    ini_Jump = 0;
    ini_time=time_sim;
    Chi_t = chi_0;
    Delta_chi = Vertical_control(des_energy,y0,y1,y1d,y2,y2d,w);
    %
    theta1_control = theta1_stance;
    %
    during:
    FY= Fy(y0,y0d);
    %
    %Chi = chi_0 + 20 * (time_sim - ini_time)^2;
    Chi = chi_0 + Delta_chi;
    Chi_t = isLower(Chi, Delta_chi);
    FK = Fk(w,wd,Chi_t);
    Chi_output=Chi_t;
    %
    [theta1_control,xTD,x2d_d] = Horizontal_control(theta2,...
    theta2_des, theta2_dot,w,x2,...
    x2d,x2_des);
    tau = Torque_flight(theta1,theta1_dot, theta1_control);
    FX =  Fx(x0,x0d,xTD);
    %
    ini_Jump = StartJump(time_sim,ini_time);
  state Touchdown_Bottom
    entry:
    theta1_control = theta1_stance;
    during:
    FY = Fy(y0,y0d);
    FK = Fk(w,wd,chi_0);
    Chi_output = chi_0;
    %
    [theta1_control,xTD,x2d_d] = Horizontal_control(theta2,...
    theta2_des, theta2_dot,w,x2,...
    x2d,x2_des);
    tau = Torque_flight(theta1,theta1_dot,...
    theta1_control);
    FX = Fx(x0,x0d,xTD);
  state Top_Touchdown
    entry:
    during:
    FY = 0;
    FX = 0;
    FK = Fk(w,wd,chi_0);
    Chi_output = chi_0;
    %Horizontal Control (Balance)
    [theta1_control,~,x2d_d] = Horizontal_control(theta2,...
    theta2_des, theta2_dot,w,x2,...
    x2d,x2_des);
    tau = Torque_stance(theta1,theta1_dot,...
    theta1_control);
  state LiftOff_Top
    entry:
    ini_time = time_sim;
    during:
    FY = 0;
    FX = 0;
    %
    %Chi = Chi_max - 13 * (time_sim - ini_time)^2;
    Chi = chi_0;
    Chi_t = isGreater(Chi, chi_0);
    FK = Fk(w,wd,Chi_t);
    Chi_output = Chi_t;
    %
    [theta1_control,~,x2d_d] = Horizontal_control(theta2,...
    theta2_des, theta2_dot,w,x2,...
    x2d,x2_des);
    tau = Torque_stance(theta1,theta1_dot,...
    theta1_control);
  Touchdown_Bottom -> Bottom_LiftOff : [wd>1.5]{theta1_stance = theta1_control;}
  Top_Touchdown -> Touchdown_Bottom : [y0<0]{theta1_stance = theta1_control;}
  Bottom_LiftOff -> LiftOff_Top : [y0>0 | ini_Jump ==1]{Chi_max = Chi_t;}
  (default) -> Top_Touchdown
  LiftOff_Top -> Top_Touchdown : [y0d<0]
  data: i_y0 function_input; output function_output; i_y0d function_input; i_des_energy function_input; i_y0 function_input; i_y1 function_input; i_y1_d function_input; i_y2 function_input; i_y2_d function_input; i_w function_input; o_chi function_output; i_x0 function_input; output function_output; i_x0d function_input; i_xTD function_input; i_Chi function_input; i_Delta_chi function_input; output function_output; i_Chi function_input; output function_output; i_Chi_min function_input; i_w function_input; output function_output; i_wd function_input; i_Chi function_input; i_time function_input; output function_output; i_ini_t function_input; i_theta2 function_input; i_theta2_des function_input; i_theta2_dot function_input; i_w function_input; i_x2 function_input; i_x2_dot function_input; o_theta1_des function_output; i_x2_des function_input; o_xTD function_output; x2_dot_des function_output; i_theta1 function_input; i_theta1_d function_input; i_theta1_des function_input; o_torque function_output; i_theta1 function_input; i_theta1_d function_input; i_theta1_des function_input; o_torque function_output; w input size=1; wd input size=1; y0 input size=1; y0d input size=1; x0 input size=1; x0d input size=1; FY output size=1; FX output size=1; FK output size=1; Chi_output output size=1; time_sim input size=1; ini_time local size=1; Chi_t local size=1; chi_0 input size=1; des_energy input size=1; y1 input size=1; y1d input size=1; y2 input size=1; y2d input size=1; Chi local size=1; Chi_max local size=1; Delta_chi local size=1; ini_Jump local size=1; theta2 input size=1; theta2_des input size=1; theta2_dot input size=1; x2 input size=1; x2d input size=1; x2_des input size=1; theta1_control output size=1; theta1_stance local size=1; theta1 input size=1; theta1_dot input size=1; tau output size=1; xTD output size=1; x2d_d output size=1
  function output = Fy(i_y0, i_y0d):
    | function output = Fy(i_y0, i_y0d)
    | KG=10^4; % [Nt/m]
    | BG=75; % [Nt-s/m]
    | output = (-KG*i_y0)-(BG*i_y0d);
  function o_chi = Vertical_control(i_des_energy,i_y0,i_y1,i_y1_d,i_y2,i_y2_d,i_w):
    | function o_chi = Vertical_control(i_des_energy,i_y0,i_y1,i_y1_d,i_y2,i_y2_d,i_w)
    | 
    | chi_min=0.05;
    | chi_max=0.18;
    | 
    | M1=1; % Leg mass [kg]
    | M2=10; % Body mass [kg]
    | 
    | k0=1; % [m]
    | KL=10^3; % [Nt/m]
    | 
    | KG=10^4; % [Nt/m]
    | g=9.8;
    | 
    | E_flight=(M2/(M1+M2))*...
    |     (M1*g*i_y1+...
    |     M2*g*i_y2+...
    |     0.5*M1*i_y1_d^2+...
    |     0.5*M2*i_y2_d^2+...
    |     0.5*(KL*(k0-i_w+0.04)^2)+...
    |     0.5*KG*i_y0^2);
    | 
    | Delta_EH=i_des_energy-E_flight;
    | 
    | Delta_chi=-(0.04-i_w+k0)+sqrt((0.04-i_w+k0)^2+((2*abs(Delta_EH))/KL));
    | 
    | if Delta_EH >= 0
    |     o_chi=chi_min+Delta_chi;
    | else
    |     o_chi=chi_min-Delta_chi;
    | end
    | 
    | if o_chi<chi_min
    |     o_chi=chi_min;
    | end
    | if o_chi>chi_max
    |     o_chi=chi_max;
    | end
  function output = Fx(i_x0, i_x0d, i_xTD):
    | function output = Fx(i_x0, i_x0d, i_xTD)
    | KG=10000; % [Nt/m]
    | BG=75; % [Nt-s/m]
    | %output = -KG*(i_x0-i_xTD )-(BG*i_x0d);
    | output = -(BG*i_x0d);
    | %output = -KG*(i_xTD )-(BG*i_x0d);
  function output = isLower (i_Chi,i_Delta_chi):
    | function output = isLower (i_Chi,i_Delta_chi)
    | 
    | if i_Chi > i_Delta_chi
    | output = i_Delta_chi;
    | else
    | output = i_Chi;
    | end
  function output = isGreater(i_Chi, i_Chi_min):
    | function output = isGreater(i_Chi, i_Chi_min)
    | 
    | if i_Chi > i_Chi_min
    | output = i_Chi;
    | else
    | output = i_Chi_min;
    | end
  function output = Fk(i_w,i_wd,i_Chi):
    | function output = Fk(i_w,i_wd,i_Chi)
    | k0=1; % [m]
    | KL=10^3; % [Nt/m]
    | 
    | KL2=60000; % [Nt/m]
    | BL2=220; % [Nt-s/m]
    | if (k0-i_w+i_Chi)>0
    |    output = KL*(k0-i_w+i_Chi);
    | else
    |     output=KL2*(k0-i_w+i_Chi)-(BL2*i_wd);
    |     if output > 0
    |         %output = 0;
    |     end
    | end
  function output = StartJump (i_time, i_ini_t):
    | function output = StartJump (i_time, i_ini_t)
    | 
    | if i_time < 1.6
    |     if (i_time - i_ini_t) > 0.4
    |         output = 1;
    |     else
    |         output = 0;
    |     end
    | else
    |     output = 0;
    | end
    | 
    | end
  function [o_theta1_des,o_xTD,x2_dot_des] = Horizontal_control(i_theta2, i_theta2_des, i_theta2_dot, i_w, i_x2, i_x2_dot, i_x2_des):
    | function [o_theta1_des,o_xTD,x2_dot_des] = Horizontal_control(i_theta2, i_theta2_des, i_theta2_dot, i_w, i_x2, i_x2_dot, i_x2_des)
    | 
    | % default params
    | M1=1; % Leg mass [kg]
    | M2=10; % Body mass [kg]
    | r1=0.5; % [m]
    | r2=0.4; % [m]
    | 
    | x2_dot_max = 1.5;
    | 
    | % choose which horizontal controller to apply
    | mode = 1;
    | 
    |     switch mode
    |         case 1
    | 
    |         % Method 1 : Foot Placement
    |         % This analysis is done in a coordinate system that translates with the hip
    | 
    |         % Control of x2 is accomplished by implementing a posisiton controller of
    |         % the form:
    |     %     x2d_dot_max = 1.5;
    |     %     K = 10;   
    |     %     x2_dot_des = min(K*(x2 - x2*1.1), x2d_dot_max);
    | 
    |         % Find Horizontal position of center of gravity
    |         %x_cg = (1/( M1+M2))*((r1-w)*M1*sin(i_theta1) + r2*M2*sin(i_theta2));
    | 
    |         % Calculate linear combination of state errors to provide corrective
    |         % feedback
    |         [K1,K2,K3] = deal(0.25, 0.06, 0.1); %(0.18, 0.06, 0.1) last:(0.25, 0.03, 0.1)
    |         %useful for position control (0.25, 0.06, 0.1)
    |         %could be for tracking (0.18, 0.20, 0.005)
    |         % x2d_dot is rechieved as input
    |         
    |         % x2d_dot is computed from (23)
    |         K=0.5;
    |         a=K*(i_x2-i_x2_des);
    |         A=[a x2_dot_max];
    |         %x2_dot_des = min(A);
    |         
    |         if a < -x2_dot_max
    |             x2_dot_des = -x2_dot_max;
    |         elseif a > x2_dot_max
    |             x2_dot_des = x2_dot_max;
    |         else
    |             x2_dot_des = a;
    |         end
    |         
    |         x_err = K1*(i_x2_dot - x2_dot_des) + K2*(i_theta2 - i_theta2_des) + K3*(i_theta2_dot);
    | 
    |         % Place foot at touchdown 
    |         %x_td = x_cg+x_err;
    | 
    |         % Foot placement wrt hip 
    |         o_xTD = i_w*( r2*M2*sin(i_theta2) + (M1+M2)*x_err)/(r1*M1 + w*M2);
    | 
    |         % The corresponding leg angle to achieve
    |         %epsi = 10^-5;
    |         argumasin = (r2*M2*sin(i_theta2) + (M1+M2)*x_err)/(r1*M1 + i_w*M2);
    |         argumasin = max(min(argumasin,1),-1);
    |         o_theta1_des = -asin(argumasin);
    |         %o_theta1_des = -asin((r2*M2*sin(i_theta2) + (M1+M2)*x_err)/(r1*M1 + i_w*M2));
    | 
    |         case 2 
    | 
    |         % Method 2 : Leg sweeping
    | 
    |         case 3
    | 
    |         % Method 3 : Servo attitude
    |     
    |     end
    | end
  function o_torque = Torque_stance(i_theta1,i_theta1_d, i_theta1_des):
    | function o_torque = Torque_stance(i_theta1,i_theta1_d, i_theta1_des)
    | 
    | Kp=1800; %[Nt-m/rad]
    | Kv=200; %[Nt-m-s/rad]
    | 
    | o_torque=Kp*(i_theta1-i_theta1_des)+Kv*(i_theta1_d);
    | 
    | end
  function o_torque = Torque_flight(i_theta1,i_theta1_d, i_theta1_des):
    | function o_torque = Torque_flight(i_theta1,i_theta1_d, i_theta1_des)
    | 
    | Kp=1200; %[Nt-m/rad]
    | Kv=60; %[Nt-m-s/rad]
    | 
    | o_torque=Kp*(i_theta1-i_theta1_des)+Kv*(i_theta1_d);
    | 
    | end
